simulink model "Sistema_Seguimiento_Tipo1_Con_Planta_Tipo_0"  (R2016a)
settings: Solver=VariableStepAuto  StartTime=0.0  StopTime=3  RelTol=1e-3
undefined symbols (not defined in the file or in its folder): A, B, C, D
settings Model: Creator=Abel  LastModifiedBy=Abel

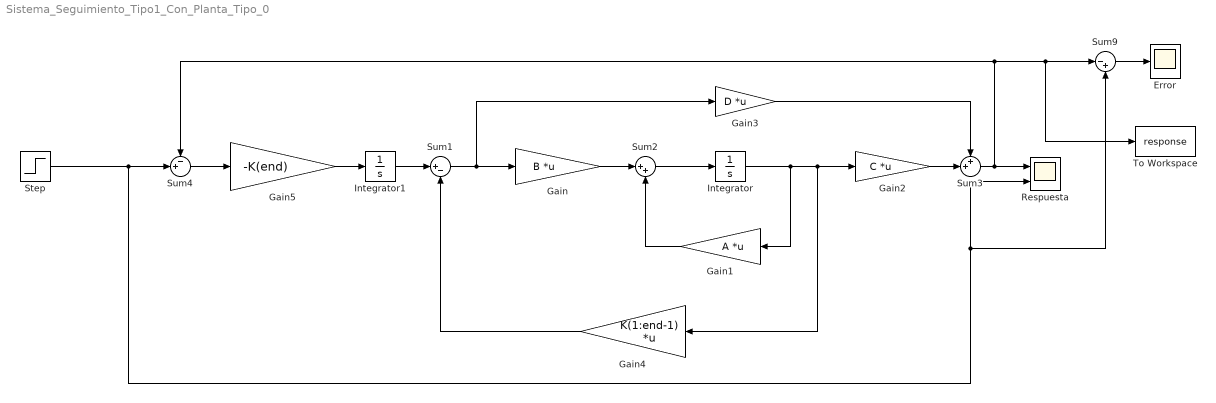
== system Sistema_Seguimiento_Tipo1_Con_Planta_Tipo_0 ==
  Error : Scope
  Gain : Gain  Gain=B  Multiplication=Matrix(K*u) (u vector)
  Gain1 : Gain  Gain=A  Multiplication=Matrix(K*u) (u vector)
  Gain2 : Gain  Gain=C  Multiplication=Matrix(K*u) (u vector)
  Gain3 : Gain  Gain=D  Multiplication=Matrix(K*u) (u vector)
  Gain4 : Gain  Gain=K(1:end-1)  Multiplication=Matrix(K*u) (u vector)
  Gain5 : Gain  Gain=-K(end)
  Integrator : Integrator
  Integrator1 : Integrator
  Respuesta : Scope  NumInputPorts=2
  Step : Step  Time=0  SampleTime=0
  Sum1 : Sum  Inputs=|+-
  Sum2 : Sum  Inputs=|++
  Sum3 : Sum  Inputs=++|
  Sum4 : Sum  Inputs=-+|
  Sum9 : Sum  Inputs=|-+
  To Workspace : ToWorkspace  VariableName=response  SaveFormat=Timeseries  SampleTime=-1
      settings: Save2DSignal=2-D array (concatenate along first dimension)
  wires:
  Sum1/1 -> Gain3/1, Gain/1
  Gain/1 -> Sum2/1
  Sum2/1 -> Integrator/1
  Gain1/1 -> Sum2/2
  Integrator/1 -> Gain4/1, Gain2/1, Gain1/1
  Gain2/1 -> Sum3/2
  Gain3/1 -> Sum3/1
  Sum3/1 -> Respuesta/1, To Workspace/1, Sum9/1, Sum4/1
  Gain4/1 -> Sum1/2
  Sum4/1 -> Gain5/1
  Step/1 -> Sum4/2, Sum9/2, Respuesta/2
  Gain5/1 -> Integrator1/1
  Integrator1/1 -> Sum1/1
  Sum9/1 -> Error/1
